simulink model "dropletdet_full"  (Simulink 8.0)
settings: Solver=ode45  StartTime=0.0  StopTime=10.0  RelTol=1e-3
undefined symbols (not defined in the file or in its folder): sfp
libraries: xbsIndex_r4 x495, dspsigops x16, xps_library x5, simulink x1, casper_library_misc x1
(part 2 of 5)

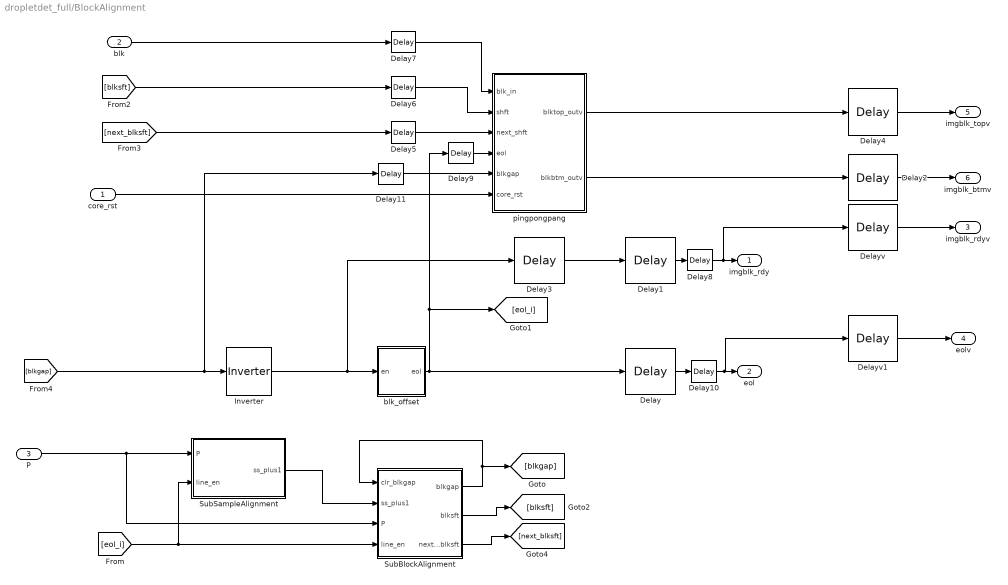
== system dropletdet_full/BlockAlignment ==
  core_rst : Inport
  blk : Inport  Port=2
  P : Inport  Port=3
  Delay{,1..4} (5 alike) : xbsIndex_r4/Delay  rst=off  infoeditControl=Selection of Reset will increase slice count due to use of real FFs and instead of SRLs  en=off  latency=1  dbl_ovrd=off  reg_retiming=off  block_type=delay
  Delay{5..11} (7 alike) : xbsIndex_r4/Delay  rst=off  infoeditControl=Selection of Reset will increase slice count due to use of real FFs and instead of SRLs  en=off  latency=4  dbl_ovrd=off  reg_retiming=off  block_type=delay
  Delayv : xbsIndex_r4/Delay  rst=off  infoeditControl=Selection of Reset will increase slice count due to use of real FFs and instead of SRLs  en=off  latency=10  dbl_ovrd=off  reg_retiming=off  block_type=delay
  Delayv1 : xbsIndex_r4/Delay  rst=off  infoeditControl=Selection of Reset will increase slice count due to use of real FFs and instead of SRLs  en=off  latency=10  dbl_ovrd=off  reg_retiming=off  block_type=delay
  Inverter : xbsIndex_r4/Inverter  en=off  latency=0  dbl_ovrd=off  block_type=inv
  SubBlockAlignment : Subsystem
  SubSampleAlignment : Subsystem
  blk_offset : Subsystem
  pingpongpang : Subsystem
  imgblk_rdy : Outport
  eol : Outport  Port=2
  imgblk_rdyv : Outport  Port=3
  eolv : Outport  Port=4
  imgblk_topv : Outport  Port=5
  imgblk_btmv : Outport  Port=6
  wires:
  SubSampleAlignment/1(ss_plus1) -> SubBlockAlignment/2(ss_plus1)
  SubBlockAlignment/1(blkgap) -> [blkgap], SubBlockAlignment/1(clr_blkgap)
  SubBlockAlignment/2(blksft) -> [blksft]
  SubBlockAlignment/3(next_blksft) -> [next_blksft]
  [eol_i] -> SubBlockAlignment/4(line_en), SubSampleAlignment/2(line_en)
  Inverter/1 -> Delay3/1, blk_offset/1(en)
  Delay4/1 -> imgblk_topv/1
  Delayv/1 -> imgblk_rdyv/1
  Delayv1/1 -> eolv/1
  [next_blksft] -> Delay5/1
  [blksft] -> Delay6/1
  [blkgap] -> Delay11/1, Inverter/1
  Delay9/1 -> pingpongpang/4(eol)
  pingpongpang/1(blktop_outv) -> Delay4/1
  Delay1/1 -> Delay8/1
  Delay/1 -> Delay10/1
  Delay3/1 -> Delay1/1
  blk_offset/1(eol) -> [eol_i], Delay9/1, Delay/1
  Delay5/1 -> pingpongpang/3(next_shft)
  Delay6/1 -> pingpongpang/2(shft)
  Delay7/1 -> pingpongpang/1(blk_in)
  Delay8/1 -> Delayv/1, imgblk_rdy/1
  Delay10/1 -> Delayv1/1, eol/1
  Delay11/1 -> pingpongpang/5(blkgap)
  P/1 -> SubBlockAlignment/3(P), SubSampleAlignment/1(P)
  blk/1 -> Delay7/1
  core_rst/1 -> pingpongpang/6(core_rst)
  pingpongpang/2(blkbtm_outv) -> Delay2/1
  Delay2/1 -> imgblk_btmv/1

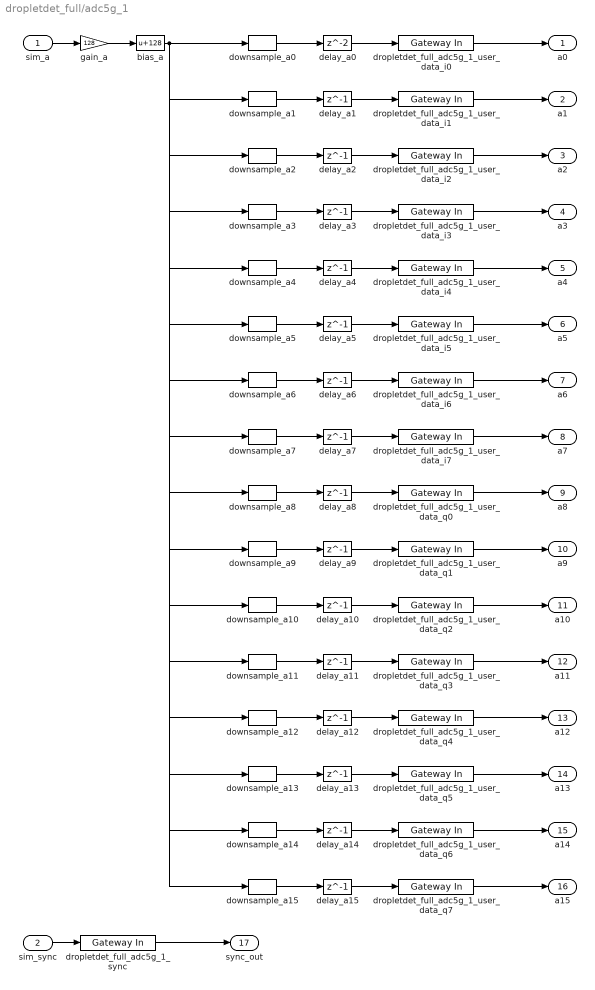
== system dropletdet_full/adc5g_1 ==
  sim_a : Inport
  sim_sync : Inport  Port=2
  bias_a : Bias  Bias=128  SaturateOnIntegerOverflow=on
  delay_a0 : Delay  InitialCondition=0  InputProcessing=Inherited
  delay_a{1..15} (15 alike) : Delay  DelayLength=1  InitialCondition=0  InputProcessing=Inherited
  downsample_a0 : dspsigops/Downsample  N=16  phase=0  RateOptions=Allow multirate processing  smode=Force single rate  fmode=Maintain input frame rate  ic=0
  downsample_a1 : dspsigops/Downsample  N=16  phase=1  RateOptions=Allow multirate processing  smode=Force single rate  fmode=Maintain input frame rate  ic=0
  downsample_a10 : dspsigops/Downsample  N=16  phase=10  RateOptions=Allow multirate processing  smode=Force single rate  fmode=Maintain input frame rate  ic=0
  downsample_a11 : dspsigops/Downsample  N=16  phase=11  RateOptions=Allow multirate processing  smode=Force single rate  fmode=Maintain input frame rate  ic=0
  downsample_a12 : dspsigops/Downsample  N=16  phase=12  RateOptions=Allow multirate processing  smode=Force single rate  fmode=Maintain input frame rate  ic=0
  downsample_a13 : dspsigops/Downsample  N=16  phase=13  RateOptions=Allow multirate processing  smode=Force single rate  fmode=Maintain input frame rate  ic=0
  downsample_a14 : dspsigops/Downsample  N=16  phase=14  RateOptions=Allow multirate processing  smode=Force single rate  fmode=Maintain input frame rate  ic=0
  downsample_a15 : dspsigops/Downsample  N=16  phase=15  RateOptions=Allow multirate processing  smode=Force single rate  fmode=Maintain input frame rate  ic=0
  downsample_a2 : dspsigops/Downsample  N=16  phase=2  RateOptions=Allow multirate processing  smode=Force single rate  fmode=Maintain input frame rate  ic=0
  downsample_a3 : dspsigops/Downsample  N=16  phase=3  RateOptions=Allow multirate processing  smode=Force single rate  fmode=Maintain input frame rate  ic=0
  downsample_a4 : dspsigops/Downsample  N=16  phase=4  RateOptions=Allow multirate processing  smode=Force single rate  fmode=Maintain input frame rate  ic=0
  downsample_a5 : dspsigops/Downsample  N=16  phase=5  RateOptions=Allow multirate processing  smode=Force single rate  fmode=Maintain input frame rate  ic=0
  downsample_a6 : dspsigops/Downsample  N=16  phase=6  RateOptions=Allow multirate processing  smode=Force single rate  fmode=Maintain input frame rate  ic=0
  downsample_a7 : dspsigops/Downsample  N=16  phase=7  RateOptions=Allow multirate processing  smode=Force single rate  fmode=Maintain input frame rate  ic=0
  downsample_a8 : dspsigops/Downsample  N=16  phase=8  RateOptions=Allow multirate processing  smode=Force single rate  fmode=Maintain input frame rate  ic=0
  downsample_a9 : dspsigops/Downsample  N=16  phase=9  RateOptions=Allow multirate processing  smode=Force single rate  fmode=Maintain input frame rate  ic=0
  dropletdet_full_adc5g_1_sync : xbsIndex_r4/Gateway In  gui_display_data_type=Fixed-point  arith_type=Boolean  n_bits=16  bin_pt=14  preci_type=Single  exp_width=8  frac_width=24  quantization="Round  (unbiased: +/- Inf)"  overflow=Saturate  period=1  dbl_ovrd=off  timing_constraint=None  locs_specified=off  LOCs={}  UseAsADC=off  ADCChannel='1'  inherit_from_input=off  hdl_port=on  block_type=gatewayin
  dropletdet_full_adc5g_1_user_data_i{0..7} (8 alike) : xbsIndex_r4/Gateway In  gui_display_data_type=Fixed-point  arith_type=Unsigned  n_bits=8  bin_pt=0  preci_type=Single  exp_width=8  frac_width=24  quantization=Truncate  overflow=Wrap  period=1  dbl_ovrd=off  timing_constraint=None  locs_specified=off  LOCs={}  UseAsADC=off  ADCChannel='1'  inherit_from_input=off  hdl_port=on  block_type=gatewayin
  dropletdet_full_adc5g_1_user_data_q{0..7} (8 alike) : xbsIndex_r4/Gateway In  gui_display_data_type=Fixed-point  arith_type=Unsigned  n_bits=8  bin_pt=0  preci_type=Single  exp_width=8  frac_width=24  quantization=Truncate  overflow=Wrap  period=1  dbl_ovrd=off  timing_constraint=None  locs_specified=off  LOCs={}  UseAsADC=off  ADCChannel='1'  inherit_from_input=off  hdl_port=on  block_type=gatewayin
  gain_a : Gain  Gain=128  SaturateOnIntegerOverflow=on  OutDataTypeStr=Inherit: Same as input  ParamDataTypeStr=Inherit: Same as input
  a0 : Outport
  a1 : Outport  Port=2
  a2 : Outport  Port=3
  a3 : Outport  Port=4
  a4 : Outport  Port=5
  a5 : Outport  Port=6
  a6 : Outport  Port=7
  a7 : Outport  Port=8
  a8 : Outport  Port=9
  a9 : Outport  Port=10
  a10 : Outport  Port=11
  a11 : Outport  Port=12
  a12 : Outport  Port=13
  a13 : Outport  Port=14
  a14 : Outport  Port=15
  a15 : Outport  Port=16
  sync_out : Outport  Port=17
  wires:
  sim_a/1 -> gain_a/1
  gain_a/1 -> bias_a/1
  bias_a/1 -> downsample_a0/1, downsample_a1/1, downsample_a2/1, downsample_a3/1, downsample_a4/1, downsample_a5/1, downsample_a6/1, downsample_a7/1, downsample_a8/1, downsample_a9/1, downsample_a10/1, downsample_a11/1, downsample_a12/1, downsample_a13/1, downsample_a14/1, downsample_a15/1
  downsample_a0/1 -> delay_a0/1
  delay_a0/1 -> dropletdet_full_adc5g_1_user_data_i0/1
  dropletdet_full_adc5g_1_user_data_i0/1 -> a0/1
  downsample_a1/1 -> delay_a1/1
  delay_a1/1 -> dropletdet_full_adc5g_1_user_data_i1/1
  dropletdet_full_adc5g_1_user_data_i1/1 -> a1/1
  downsample_a2/1 -> delay_a2/1
  delay_a2/1 -> dropletdet_full_adc5g_1_user_data_i2/1
  dropletdet_full_adc5g_1_user_data_i2/1 -> a2/1
  downsample_a3/1 -> delay_a3/1
  delay_a3/1 -> dropletdet_full_adc5g_1_user_data_i3/1
  dropletdet_full_adc5g_1_user_data_i3/1 -> a3/1
  downsample_a4/1 -> delay_a4/1
  delay_a4/1 -> dropletdet_full_adc5g_1_user_data_i4/1
  dropletdet_full_adc5g_1_user_data_i4/1 -> a4/1
  downsample_a5/1 -> delay_a5/1
  delay_a5/1 -> dropletdet_full_adc5g_1_user_data_i5/1
  dropletdet_full_adc5g_1_user_data_i5/1 -> a5/1
  downsample_a6/1 -> delay_a6/1
  delay_a6/1 -> dropletdet_full_adc5g_1_user_data_i6/1
  dropletdet_full_adc5g_1_user_data_i6/1 -> a6/1
  downsample_a7/1 -> delay_a7/1
  delay_a7/1 -> dropletdet_full_adc5g_1_user_data_i7/1
  dropletdet_full_adc5g_1_user_data_i7/1 -> a7/1
  downsample_a8/1 -> delay_a8/1
  delay_a8/1 -> dropletdet_full_adc5g_1_user_data_q0/1
  dropletdet_full_adc5g_1_user_data_q0/1 -> a8/1
  downsample_a9/1 -> delay_a9/1
  delay_a9/1 -> dropletdet_full_adc5g_1_user_data_q1/1
  dropletdet_full_adc5g_1_user_data_q1/1 -> a9/1
  downsample_a10/1 -> delay_a10/1
  delay_a10/1 -> dropletdet_full_adc5g_1_user_data_q2/1
  dropletdet_full_adc5g_1_user_data_q2/1 -> a10/1
  downsample_a11/1 -> delay_a11/1
  delay_a11/1 -> dropletdet_full_adc5g_1_user_data_q3/1
  dropletdet_full_adc5g_1_user_data_q3/1 -> a11/1
  downsample_a12/1 -> delay_a12/1
  delay_a12/1 -> dropletdet_full_adc5g_1_user_data_q4/1
  dropletdet_full_adc5g_1_user_data_q4/1 -> a12/1
  downsample_a13/1 -> delay_a13/1
  delay_a13/1 -> dropletdet_full_adc5g_1_user_data_q5/1
  dropletdet_full_adc5g_1_user_data_q5/1 -> a13/1
  downsample_a14/1 -> delay_a14/1
  delay_a14/1 -> dropletdet_full_adc5g_1_user_data_q6/1
  dropletdet_full_adc5g_1_user_data_q6/1 -> a14/1
  downsample_a15/1 -> delay_a15/1
  delay_a15/1 -> dropletdet_full_adc5g_1_user_data_q7/1
  dropletdet_full_adc5g_1_user_data_q7/1 -> a15/1
  sim_sync/1 -> dropletdet_full_adc5g_1_sync/1
  dropletdet_full_adc5g_1_sync/1 -> sync_out/1

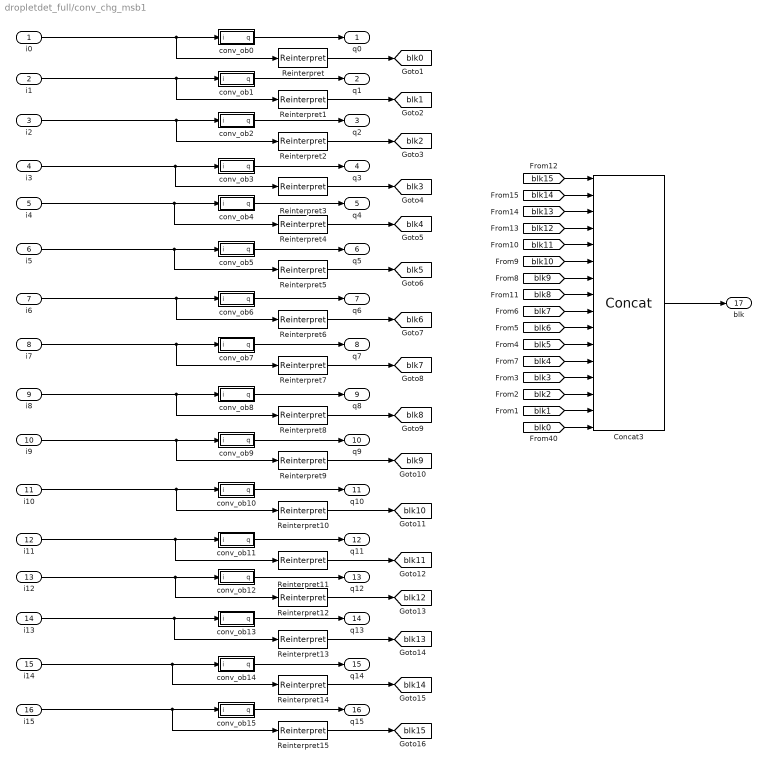
== system dropletdet_full/conv_chg_msb1 ==
  i0 : Inport
  i1 : Inport  Port=2
  i2 : Inport  Port=3
  i3 : Inport  Port=4
  i4 : Inport  Port=5
  i5 : Inport  Port=6
  i6 : Inport  Port=7
  i7 : Inport  Port=8
  i8 : Inport  Port=9
  i9 : Inport  Port=10
  i10 : Inport  Port=11
  i11 : Inport  Port=12
  i12 : Inport  Port=13
  i13 : Inport  Port=14
  i14 : Inport  Port=15
  i15 : Inport  Port=16
  Concat3 : xbsIndex_r4/Concat  num_inputs=16  dbl_ovrd=off  block_type=concat
  Reinterpret{,1..15} (16 alike) : xbsIndex_r4/Reinterpret  force_arith_type=on  arith_type=Unsigned  force_bin_pt=on  bin_pt=0  block_type=reinterpret
  conv_ob0 : Subsystem
  conv_ob1 : Subsystem
  conv_ob10 : Subsystem
  conv_ob11 : Subsystem
  conv_ob12 : Subsystem
  conv_ob13 : Subsystem
  conv_ob14 : Subsystem
  conv_ob15 : Subsystem
  conv_ob2 : Subsystem
  conv_ob3 : Subsystem
  conv_ob4 : Subsystem
  conv_ob5 : Subsystem
  conv_ob6 : Subsystem
  conv_ob7 : Subsystem
  conv_ob8 : Subsystem
  conv_ob9 : Subsystem
  q0 : Outport
  q1 : Outport  Port=2
  q2 : Outport  Port=3
  q3 : Outport  Port=4
  q4 : Outport  Port=5
  q5 : Outport  Port=6
  q6 : Outport  Port=7
  q7 : Outport  Port=8
  q8 : Outport  Port=9
  q9 : Outport  Port=10
  q10 : Outport  Port=11
  q11 : Outport  Port=12
  q12 : Outport  Port=13
  q13 : Outport  Port=14
  q14 : Outport  Port=15
  q15 : Outport  Port=16
  blk : Outport  Port=17
  tag scope: blk0=global, blk10=global, blk11=global, blk12=global, blk13=global, blk14=global, blk15=global, blk1=global, blk2=global, blk3=global, blk4=global, blk5=global, blk6=global, blk7=global, blk8=global, blk9=global
  wires:
  conv_ob15/1(q) -> q15/1
  conv_ob14/1(q) -> q14/1
  conv_ob13/1(q) -> q13/1
  conv_ob12/1(q) -> q12/1
  conv_ob11/1(q) -> q11/1
  conv_ob10/1(q) -> q10/1
  conv_ob9/1(q) -> q9/1
  conv_ob8/1(q) -> q8/1
  conv_ob7/1(q) -> q7/1
  conv_ob6/1(q) -> q6/1
  conv_ob5/1(q) -> q5/1
  conv_ob4/1(q) -> q4/1
  conv_ob3/1(q) -> q3/1
  conv_ob2/1(q) -> q2/1
  conv_ob1/1(q) -> q1/1
  conv_ob0/1(q) -> q0/1
  i0/1 -> Reinterpret/1, conv_ob0/1(i)
  i1/1 -> Reinterpret1/1, conv_ob1/1(i)
  i2/1 -> Reinterpret2/1, conv_ob2/1(i)
  i3/1 -> Reinterpret3/1, conv_ob3/1(i)
  Reinterpret/1 -> [blk0]
  Reinterpret1/1 -> [blk1]
  Reinterpret2/1 -> [blk2]
  Reinterpret3/1 -> [blk3]
  i4/1 -> Reinterpret4/1, conv_ob4/1(i)
  Reinterpret4/1 -> [blk4]
  i5/1 -> Reinterpret5/1, conv_ob5/1(i)
  Reinterpret5/1 -> [blk5]
  i6/1 -> Reinterpret6/1, conv_ob6/1(i)
  Reinterpret6/1 -> [blk6]
  i7/1 -> Reinterpret7/1, conv_ob7/1(i)
  Reinterpret7/1 -> [blk7]
  i8/1 -> Reinterpret8/1, conv_ob8/1(i)
  Reinterpret8/1 -> [blk8]
  i9/1 -> Reinterpret9/1, conv_ob9/1(i)
  Reinterpret9/1 -> [blk9]
  i10/1 -> Reinterpret10/1, conv_ob10/1(i)
  Reinterpret10/1 -> [blk10]
  i11/1 -> Reinterpret11/1, conv_ob11/1(i)
  Reinterpret11/1 -> [blk11]
  i12/1 -> Reinterpret12/1, conv_ob12/1(i)
  Reinterpret12/1 -> [blk12]
  i13/1 -> Reinterpret13/1, conv_ob13/1(i)
  Reinterpret13/1 -> [blk13]
  i14/1 -> Reinterpret14/1, conv_ob14/1(i)
  Reinterpret14/1 -> [blk14]
  i15/1 -> Reinterpret15/1, conv_ob15/1(i)
  Reinterpret15/1 -> [blk15]
  [blk10] -> Concat3/6
  [blk9] -> Concat3/7
  [blk1] -> Concat3/15
  [blk11] -> Concat3/5
  [blk7] -> Concat3/9
  [blk8] -> Concat3/8
  [blk15] -> Concat3/1
  [blk12] -> Concat3/4
  [blk13] -> Concat3/3
  [blk14] -> Concat3/2
  [blk2] -> Concat3/14
  [blk3] -> Concat3/13
  [blk5] -> Concat3/11
  [blk0] -> Concat3/16
  [blk6] -> Concat3/10
  [blk4] -> Concat3/12
  Concat3/1 -> blk/1

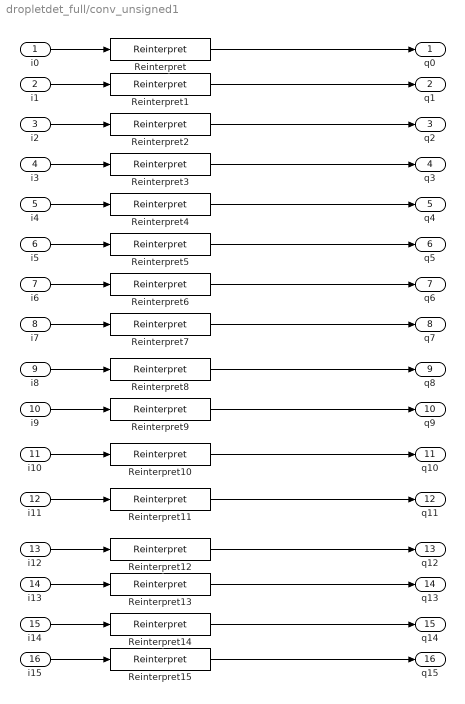
== system dropletdet_full/conv_unsigned1 ==
  i0 : Inport
  i1 : Inport  Port=2
  i2 : Inport  Port=3
  i3 : Inport  Port=4
  i4 : Inport  Port=5
  i5 : Inport  Port=6
  i6 : Inport  Port=7
  i7 : Inport  Port=8
  i8 : Inport  Port=9
  i9 : Inport  Port=10
  i10 : Inport  Port=11
  i11 : Inport  Port=12
  i12 : Inport  Port=13
  i13 : Inport  Port=14
  i14 : Inport  Port=15
  i15 : Inport  Port=16
  Reinterpret{,1..15} (16 alike) : xbsIndex_r4/Reinterpret  force_arith_type=on  arith_type=Unsigned  force_bin_pt=on  bin_pt=0  block_type=reinterpret
  q0 : Outport
  q1 : Outport  Port=2
  q2 : Outport  Port=3
  q3 : Outport  Port=4
  q4 : Outport  Port=5
  q5 : Outport  Port=6
  q6 : Outport  Port=7
  q7 : Outport  Port=8
  q8 : Outport  Port=9
  q9 : Outport  Port=10
  q10 : Outport  Port=11
  q11 : Outport  Port=12
  q12 : Outport  Port=13
  q13 : Outport  Port=14
  q14 : Outport  Port=15
  q15 : Outport  Port=16
  wires:
  i0/1 -> Reinterpret/1
  Reinterpret/1 -> q0/1
  i1/1 -> Reinterpret1/1
  Reinterpret1/1 -> q1/1
  i2/1 -> Reinterpret2/1
  Reinterpret2/1 -> q2/1
  i3/1 -> Reinterpret3/1
  i4/1 -> Reinterpret4/1
  i5/1 -> Reinterpret5/1
  i6/1 -> Reinterpret6/1
  i7/1 -> Reinterpret7/1
  i8/1 -> Reinterpret8/1
  i9/1 -> Reinterpret9/1
  i10/1 -> Reinterpret10/1
  Reinterpret3/1 -> q3/1
  Reinterpret4/1 -> q4/1
  Reinterpret5/1 -> q5/1
  Reinterpret6/1 -> q6/1
  Reinterpret7/1 -> q7/1
  Reinterpret8/1 -> q8/1
  Reinterpret9/1 -> q9/1
  Reinterpret10/1 -> q10/1
  i11/1 -> Reinterpret11/1
  Reinterpret11/1 -> q11/1
  i12/1 -> Reinterpret12/1
  Reinterpret12/1 -> q12/1
  i13/1 -> Reinterpret13/1
  Reinterpret13/1 -> q13/1
  i14/1 -> Reinterpret14/1
  Reinterpret14/1 -> q14/1
  i15/1 -> Reinterpret15/1
  Reinterpret15/1 -> q15/1

== system dropletdet_full/dealy3pipe ==
  d : Inport
  Register0 : xbsIndex_r4/Register  init=0  rst=off  en=off  dbl_ovrd=off  block_type=register
      settings: block_version=11.4
  Register1 : xbsIndex_r4/Register  init=0  rst=off  en=off  dbl_ovrd=off  block_type=register
      settings: block_version=11.4
  Register2 : xbsIndex_r4/Register  init=0  rst=off  en=off  dbl_ovrd=off  block_type=register
      settings: block_version=11.4
  q : Outport
  wires:
  Register0/1 -> Register1/1
  Register1/1 -> Register2/1
  d/1 -> Register0/1
  Register2/1 -> q/1

== system dropletdet_full/dealy3pipe1 ==
  d : Inport
  Register0 : xbsIndex_r4/Register  init=0  rst=off  en=off  dbl_ovrd=off  block_type=register
      settings: block_version=11.4
  Register1 : xbsIndex_r4/Register  init=0  rst=off  en=off  dbl_ovrd=off  block_type=register
      settings: block_version=11.4
  Register2 : xbsIndex_r4/Register  init=0  rst=off  en=off  dbl_ovrd=off  block_type=register
      settings: block_version=11.4
  q : Outport
  wires:
  Register0/1 -> Register1/1
  Register1/1 -> Register2/1
  d/1 -> Register0/1
  Register2/1 -> q/1

== system dropletdet_full/dealy3pipe2 ==
  d : Inport
  Register0 : xbsIndex_r4/Register  init=0  rst=off  en=off  dbl_ovrd=off  block_type=register
      settings: block_version=11.4
  Register1 : xbsIndex_r4/Register  init=0  rst=off  en=off  dbl_ovrd=off  block_type=register
      settings: block_version=11.4
  Register2 : xbsIndex_r4/Register  init=0  rst=off  en=off  dbl_ovrd=off  block_type=register
      settings: block_version=11.4
  q : Outport
  wires:
  Register0/1 -> Register1/1
  Register1/1 -> Register2/1
  d/1 -> Register0/1
  Register2/1 -> q/1

== system dropletdet_full/dest_ip0 ==
  sim_1 : Inport
  dropletdet_full_dest_ip0_user_data_out : xbsIndex_r4/Gateway In  gui_display_data_type=Fixed-point  arith_type=Unsigned  n_bits=32  bin_pt=0  preci_type=Single  exp_width=8  frac_width=24  quantization="Round  (unbiased: +/- Inf)"  overflow=Saturate  period=1  dbl_ovrd=off  timing_constraint=None  locs_specified=off  LOCs={}  UseAsADC=off  ADCChannel='1'  inherit_from_input=off  hdl_port=on  block_type=gatewayin
  io_delay : xbsIndex_r4/Delay  rst=off  infoeditControl=Selection of Reset will increase slice count due to use of real FFs and instead of SRLs  en=off  latency=0  dbl_ovrd=off  reg_retiming=on  block_type=delay
  reint1 : xbsIndex_r4/Reinterpret  force_arith_type=on  arith_type=Unsigned  force_bin_pt=on  bin_pt=0  block_type=reinterpret
  slice_reg : xbsIndex_r4/Slice  nbits=32  boolean_output=off  mode=Lower Bit Location + Width  bit1=0  base1=MSB of Input  bit0=0  base0=LSB of Input  dbl_ovrd=off  block_type=slice
  in_reg : Outport
  wires:
  dropletdet_full_dest_ip0_user_data_out/1 -> io_delay/1
  sim_1/1 -> dropletdet_full_dest_ip0_user_data_out/1
  io_delay/1 -> slice_reg/1
  slice_reg/1 -> reint1/1
  reint1/1 -> in_reg/1

== system dropletdet_full/dest_ip1 ==
  sim_1 : Inport
  dropletdet_full_dest_ip1_user_data_out : xbsIndex_r4/Gateway In  gui_display_data_type=Fixed-point  arith_type=Unsigned  n_bits=32  bin_pt=0  preci_type=Single  exp_width=8  frac_width=24  quantization="Round  (unbiased: +/- Inf)"  overflow=Saturate  period=1  dbl_ovrd=off  timing_constraint=None  locs_specified=off  LOCs={}  UseAsADC=off  ADCChannel='1'  inherit_from_input=off  hdl_port=on  block_type=gatewayin
  io_delay : xbsIndex_r4/Delay  rst=off  infoeditControl=Selection of Reset will increase slice count due to use of real FFs and instead of SRLs  en=off  latency=0  dbl_ovrd=off  reg_retiming=on  block_type=delay
  reint1 : xbsIndex_r4/Reinterpret  force_arith_type=on  arith_type=Unsigned  force_bin_pt=on  bin_pt=0  block_type=reinterpret
  slice_reg : xbsIndex_r4/Slice  nbits=32  boolean_output=off  mode=Lower Bit Location + Width  bit1=0  base1=MSB of Input  bit0=0  base0=LSB of Input  dbl_ovrd=off  block_type=slice
  in_reg : Outport
  wires:
  dropletdet_full_dest_ip1_user_data_out/1 -> io_delay/1
  sim_1/1 -> dropletdet_full_dest_ip1_user_data_out/1
  io_delay/1 -> slice_reg/1
  slice_reg/1 -> reint1/1
  reint1/1 -> in_reg/1

== system dropletdet_full/dest_ip2 ==
  sim_1 : Inport
  dropletdet_full_dest_ip2_user_data_out : xbsIndex_r4/Gateway In  gui_display_data_type=Fixed-point  arith_type=Unsigned  n_bits=32  bin_pt=0  preci_type=Single  exp_width=8  frac_width=24  quantization="Round  (unbiased: +/- Inf)"  overflow=Saturate  period=1  dbl_ovrd=off  timing_constraint=None  locs_specified=off  LOCs={}  UseAsADC=off  ADCChannel='1'  inherit_from_input=off  hdl_port=on  block_type=gatewayin
  io_delay : xbsIndex_r4/Delay  rst=off  infoeditControl=Selection of Reset will increase slice count due to use of real FFs and instead of SRLs  en=off  latency=0  dbl_ovrd=off  reg_retiming=on  block_type=delay
  reint1 : xbsIndex_r4/Reinterpret  force_arith_type=on  arith_type=Unsigned  force_bin_pt=on  bin_pt=0  block_type=reinterpret
  slice_reg : xbsIndex_r4/Slice  nbits=32  boolean_output=off  mode=Lower Bit Location + Width  bit1=0  base1=MSB of Input  bit0=0  base0=LSB of Input  dbl_ovrd=off  block_type=slice
  in_reg : Outport
  wires:
  dropletdet_full_dest_ip2_user_data_out/1 -> io_delay/1
  sim_1/1 -> dropletdet_full_dest_ip2_user_data_out/1
  io_delay/1 -> slice_reg/1
  slice_reg/1 -> reint1/1
  reint1/1 -> in_reg/1

== system dropletdet_full/dest_ip3 ==
  sim_1 : Inport
  dropletdet_full_dest_ip3_user_data_out : xbsIndex_r4/Gateway In  gui_display_data_type=Fixed-point  arith_type=Unsigned  n_bits=32  bin_pt=0  preci_type=Single  exp_width=8  frac_width=24  quantization="Round  (unbiased: +/- Inf)"  overflow=Saturate  period=1  dbl_ovrd=off  timing_constraint=None  locs_specified=off  LOCs={}  UseAsADC=off  ADCChannel='1'  inherit_from_input=off  hdl_port=on  block_type=gatewayin
  io_delay : xbsIndex_r4/Delay  rst=off  infoeditControl=Selection of Reset will increase slice count due to use of real FFs and instead of SRLs  en=off  latency=0  dbl_ovrd=off  reg_retiming=on  block_type=delay
  reint1 : xbsIndex_r4/Reinterpret  force_arith_type=on  arith_type=Unsigned  force_bin_pt=on  bin_pt=0  block_type=reinterpret
  slice_reg : xbsIndex_r4/Slice  nbits=32  boolean_output=off  mode=Lower Bit Location + Width  bit1=0  base1=MSB of Input  bit0=0  base0=LSB of Input  dbl_ovrd=off  block_type=slice
  in_reg : Outport
  wires:
  dropletdet_full_dest_ip3_user_data_out/1 -> io_delay/1
  sim_1/1 -> dropletdet_full_dest_ip3_user_data_out/1
  io_delay/1 -> slice_reg/1
  slice_reg/1 -> reint1/1
  reint1/1 -> in_reg/1

== system dropletdet_full/dest_port0 ==
  sim_1 : Inport
  dropletdet_full_dest_port0_user_data_out : xbsIndex_r4/Gateway In  gui_display_data_type=Fixed-point  arith_type=Unsigned  n_bits=32  bin_pt=0  preci_type=Single  exp_width=8  frac_width=24  quantization="Round  (unbiased: +/- Inf)"  overflow=Saturate  period=1  dbl_ovrd=off  timing_constraint=None  locs_specified=off  LOCs={}  UseAsADC=off  ADCChannel='1'  inherit_from_input=off  hdl_port=on  block_type=gatewayin
  io_delay : xbsIndex_r4/Delay  rst=off  infoeditControl=Selection of Reset will increase slice count due to use of real FFs and instead of SRLs  en=off  latency=0  dbl_ovrd=off  reg_retiming=on  block_type=delay
  reint1 : xbsIndex_r4/Reinterpret  force_arith_type=on  arith_type=Unsigned  force_bin_pt=on  bin_pt=0  block_type=reinterpret
  slice_reg : xbsIndex_r4/Slice  nbits=32  boolean_output=off  mode=Lower Bit Location + Width  bit1=0  base1=MSB of Input  bit0=0  base0=LSB of Input  dbl_ovrd=off  block_type=slice
  in_reg : Outport
  wires:
  dropletdet_full_dest_port0_user_data_out/1 -> io_delay/1
  sim_1/1 -> dropletdet_full_dest_port0_user_data_out/1
  io_delay/1 -> slice_reg/1
  slice_reg/1 -> reint1/1
  reint1/1 -> in_reg/1

== system dropletdet_full/dest_port1 ==
  sim_1 : Inport
  dropletdet_full_dest_port1_user_data_out : xbsIndex_r4/Gateway In  gui_display_data_type=Fixed-point  arith_type=Unsigned  n_bits=32  bin_pt=0  preci_type=Single  exp_width=8  frac_width=24  quantization="Round  (unbiased: +/- Inf)"  overflow=Saturate  period=1  dbl_ovrd=off  timing_constraint=None  locs_specified=off  LOCs={}  UseAsADC=off  ADCChannel='1'  inherit_from_input=off  hdl_port=on  block_type=gatewayin
  io_delay : xbsIndex_r4/Delay  rst=off  infoeditControl=Selection of Reset will increase slice count due to use of real FFs and instead of SRLs  en=off  latency=0  dbl_ovrd=off  reg_retiming=on  block_type=delay
  reint1 : xbsIndex_r4/Reinterpret  force_arith_type=on  arith_type=Unsigned  force_bin_pt=on  bin_pt=0  block_type=reinterpret
  slice_reg : xbsIndex_r4/Slice  nbits=32  boolean_output=off  mode=Lower Bit Location + Width  bit1=0  base1=MSB of Input  bit0=0  base0=LSB of Input  dbl_ovrd=off  block_type=slice
  in_reg : Outport
  wires:
  dropletdet_full_dest_port1_user_data_out/1 -> io_delay/1
  sim_1/1 -> dropletdet_full_dest_port1_user_data_out/1
  io_delay/1 -> slice_reg/1
  slice_reg/1 -> reint1/1
  reint1/1 -> in_reg/1

== system dropletdet_full/dest_port2 ==
  sim_1 : Inport
  dropletdet_full_dest_port2_user_data_out : xbsIndex_r4/Gateway In  gui_display_data_type=Fixed-point  arith_type=Unsigned  n_bits=32  bin_pt=0  preci_type=Single  exp_width=8  frac_width=24  quantization="Round  (unbiased: +/- Inf)"  overflow=Saturate  period=1  dbl_ovrd=off  timing_constraint=None  locs_specified=off  LOCs={}  UseAsADC=off  ADCChannel='1'  inherit_from_input=off  hdl_port=on  block_type=gatewayin
  io_delay : xbsIndex_r4/Delay  rst=off  infoeditControl=Selection of Reset will increase slice count due to use of real FFs and instead of SRLs  en=off  latency=0  dbl_ovrd=off  reg_retiming=on  block_type=delay
  reint1 : xbsIndex_r4/Reinterpret  force_arith_type=on  arith_type=Unsigned  force_bin_pt=on  bin_pt=0  block_type=reinterpret
  slice_reg : xbsIndex_r4/Slice  nbits=32  boolean_output=off  mode=Lower Bit Location + Width  bit1=0  base1=MSB of Input  bit0=0  base0=LSB of Input  dbl_ovrd=off  block_type=slice
  in_reg : Outport
  wires:
  dropletdet_full_dest_port2_user_data_out/1 -> io_delay/1
  sim_1/1 -> dropletdet_full_dest_port2_user_data_out/1
  io_delay/1 -> slice_reg/1
  slice_reg/1 -> reint1/1
  reint1/1 -> in_reg/1

== system dropletdet_full/dest_port3 ==
  sim_1 : Inport
  dropletdet_full_dest_port3_user_data_out : xbsIndex_r4/Gateway In  gui_display_data_type=Fixed-point  arith_type=Unsigned  n_bits=32  bin_pt=0  preci_type=Single  exp_width=8  frac_width=24  quantization="Round  (unbiased: +/- Inf)"  overflow=Saturate  period=1  dbl_ovrd=off  timing_constraint=None  locs_specified=off  LOCs={}  UseAsADC=off  ADCChannel='1'  inherit_from_input=off  hdl_port=on  block_type=gatewayin
  io_delay : xbsIndex_r4/Delay  rst=off  infoeditControl=Selection of Reset will increase slice count due to use of real FFs and instead of SRLs  en=off  latency=0  dbl_ovrd=off  reg_retiming=on  block_type=delay
  reint1 : xbsIndex_r4/Reinterpret  force_arith_type=on  arith_type=Unsigned  force_bin_pt=on  bin_pt=0  block_type=reinterpret
  slice_reg : xbsIndex_r4/Slice  nbits=32  boolean_output=off  mode=Lower Bit Location + Width  bit1=0  base1=MSB of Input  bit0=0  base0=LSB of Input  dbl_ovrd=off  block_type=slice
  in_reg : Outport
  wires:
  dropletdet_full_dest_port3_user_data_out/1 -> io_delay/1
  sim_1/1 -> dropletdet_full_dest_port3_user_data_out/1
  io_delay/1 -> slice_reg/1
  slice_reg/1 -> reint1/1
  reint1/1 -> in_reg/1

== system dropletdet_full/enable ==
  sim_1 : Inport
  dropletdet_full_enable_user_data_out : xbsIndex_r4/Gateway In  gui_display_data_type=Fixed-point  arith_type=Unsigned  n_bits=32  bin_pt=0  preci_type=Single  exp_width=8  frac_width=24  quantization="Round  (unbiased: +/- Inf)"  overflow=Saturate  period=1  dbl_ovrd=off  timing_constraint=None  locs_specified=off  LOCs={}  UseAsADC=off  ADCChannel='1'  inherit_from_input=off  hdl_port=on  block_type=gatewayin
  io_delay : xbsIndex_r4/Delay  rst=off  infoeditControl=Selection of Reset will increase slice count due to use of real FFs and instead of SRLs  en=off  latency=0  dbl_ovrd=off  reg_retiming=on  block_type=delay
  reint1 : xbsIndex_r4/Reinterpret  force_arith_type=on  arith_type=Unsigned  force_bin_pt=on  bin_pt=0  block_type=reinterpret
  slice_reg : xbsIndex_r4/Slice  nbits=32  boolean_output=off  mode=Lower Bit Location + Width  bit1=0  base1=MSB of Input  bit0=0  base0=LSB of Input  dbl_ovrd=off  block_type=slice
  in_reg : Outport
  wires:
  dropletdet_full_enable_user_data_out/1 -> io_delay/1
  sim_1/1 -> dropletdet_full_enable_user_data_out/1
  io_delay/1 -> slice_reg/1
  slice_reg/1 -> reint1/1
  reint1/1 -> in_reg/1

== system dropletdet_full/period ==
  sim_1 : Inport
  dropletdet_full_period_user_data_out : xbsIndex_r4/Gateway In  gui_display_data_type=Fixed-point  arith_type=Unsigned  n_bits=32  bin_pt=0  preci_type=Single  exp_width=8  frac_width=24  quantization="Round  (unbiased: +/- Inf)"  overflow=Saturate  period=1  dbl_ovrd=off  timing_constraint=None  locs_specified=off  LOCs={}  UseAsADC=off  ADCChannel='1'  inherit_from_input=off  hdl_port=on  block_type=gatewayin
  io_delay : xbsIndex_r4/Delay  rst=off  infoeditControl=Selection of Reset will increase slice count due to use of real FFs and instead of SRLs  en=off  latency=0  dbl_ovrd=off  reg_retiming=on  block_type=delay
  reint1 : xbsIndex_r4/Reinterpret  force_arith_type=on  arith_type="Signed  (2's comp)"  force_bin_pt=on  bin_pt=20  block_type=reinterpret
  slice_period : xbsIndex_r4/Slice  nbits=32  boolean_output=off  mode=Lower Bit Location + Width  bit1=0  base1=MSB of Input  bit0=0  base0=LSB of Input  dbl_ovrd=off  block_type=slice
  in_period : Outport
  wires:
  dropletdet_full_period_user_data_out/1 -> io_delay/1
  sim_1/1 -> dropletdet_full_period_user_data_out/1
  io_delay/1 -> slice_period/1
  slice_period/1 -> reint1/1
  reint1/1 -> in_period/1
